simulink library "STMM"  (R2024a)
settings: Solver=VariableStepAuto  StartTime=0.0  StopTime=10.0  RelTol=1e-3
undefined symbols (not defined in the file or in its folder): raptor_xcp_function, StateCAN
libraries: Utilities x260, Raptor_lib x68, simulink x2
(part 3 of 3)

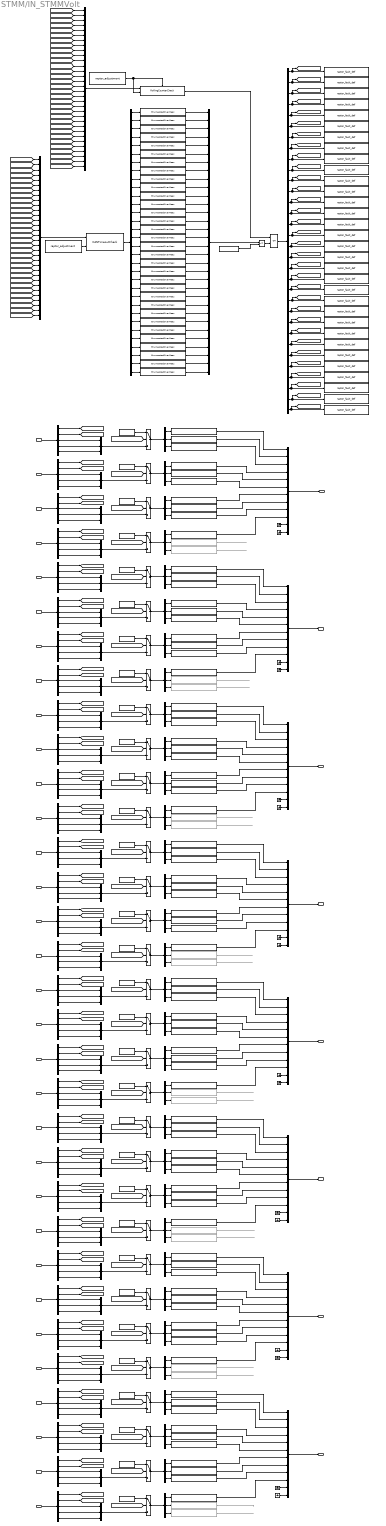
== system STMM/IN_STMMVolt ==
  IO_CAN2_332_Bus : Inport
  IO_CAN2_333_Bus : Inport  Port=2
  IO_CAN2_334_Bus : Inport  Port=3
  IO_CAN2_335_Bus : Inport  Port=4
  IO_CAN2_336_Bus : Inport  Port=5
  IO_CAN2_337_Bus : Inport  Port=6
  IO_CAN2_338_Bus : Inport  Port=7
  IO_CAN2_339_Bus : Inport  Port=8
  IO_CAN2_340_Bus : Inport  Port=9
  IO_CAN2_341_Bus : Inport  Port=10
  IO_CAN2_342_Bus : Inport  Port=11
  IO_CAN2_343_Bus : Inport  Port=12
  IO_CAN2_344_Bus : Inport  Port=13
  IO_CAN2_345_Bus : Inport  Port=14
  IO_CAN2_346_Bus : Inport  Port=15
  IO_CAN2_347_Bus : Inport  Port=16
  IO_CAN2_348_Bus : Inport  Port=17
  IO_CAN2_349_Bus : Inport  Port=18
  IO_CAN2_350_Bus : Inport  Port=19
  IO_CAN2_351_Bus : Inport  Port=20
  IO_CAN2_352_Bus : Inport  Port=21
  IO_CAN2_353_Bus : Inport  Port=22
  IO_CAN2_354_Bus : Inport  Port=23
  IO_CAN2_355_Bus : Inport  Port=24
  IO_CAN2_356_Bus : Inport  Port=25
  IO_CAN2_357_Bus : Inport  Port=26
  IO_CAN2_358_Bus : Inport  Port=27
  IO_CAN2_359_Bus : Inport  Port=28
  IO_CAN2_360_Bus : Inport  Port=29
  IO_CAN2_361_Bus : Inport  Port=30
  IO_CAN2_362_Bus : Inport  Port=31
  IO_CAN2_363_Bus : Inport  Port=32
  Bus Creator{,1..7} (8 alike) : BusCreator  Inputs=12
  Bus Selector : BusSelector  OutputSignals=Age,STMM_counterMsg332,STMM_segmentVolt100,STMM_segmentVolt101,STMM_segmentVolt102
  Bus Selector1 : BusSelector  OutputSignals=Age,STMM_counterMsg333,STMM_segmentVolt103,STMM_segmentVolt104,STMM_segmentVolt105
  Bus Selector10 : BusSelector  OutputSignals=Age,STMM_counterMsg342,STMM_segmentVolt306,STMM_segmentVolt307,STMM_segmentVolt308
  Bus Selector11 : BusSelector  OutputSignals=Age,STMM_counterMsg343,STMM_segmentVolt309,STMM_segmentVolt310,STMM_segmentVolt311
  Bus Selector12 : BusSelector  OutputSignals=Age,STMM_counterMsg344,STMM_segmentVolt400,STMM_segmentVolt401,STMM_segmentVolt402
  Bus Selector13 : BusSelector  OutputSignals=Age,STMM_counterMsg345,STMM_segmentVolt403,STMM_segmentVolt404,STMM_segmentVolt405
  Bus Selector14 : BusSelector  OutputSignals=Age,STMM_counterMsg346,STMM_segmentVolt406,STMM_segmentVolt407,STMM_segmentVolt408
  Bus Selector15 : BusSelector  OutputSignals=Age,STMM_counterMsg347,STMM_segmentVolt409,STMM_segmentVolt410,STMM_segmentVolt411
  Bus Selector16 : BusSelector  OutputSignals=Age,STMM_counterMsg348,STMM_segmentVolt500,STMM_segmentVolt501,STMM_segmentVolt502
  Bus Selector17 : BusSelector  OutputSignals=Age,STMM_counterMsg349,STMM_segmentVolt503,STMM_segmentVolt504,STMM_segmentVolt505
  Bus Selector18 : BusSelector  OutputSignals=Age,STMM_counterMsg350,STMM_segmentVolt506,STMM_segmentVolt507,STMM_segmentVolt508
  Bus Selector19 : BusSelector  OutputSignals=Age,STMM_counterMsg351,STMM_segmentVolt509,STMM_segmentVolt510,STMM_segmentVolt511
  Bus Selector2 : BusSelector  OutputSignals=Age,STMM_counterMsg334,STMM_segmentVolt106,STMM_segmentVolt107,STMM_segmentVolt108
  Bus Selector20 : BusSelector  OutputSignals=Age,STMM_counterMsg352,STMM_segmentVolt600,STMM_segmentVolt601,STMM_segmentVolt602
  Bus Selector21 : BusSelector  OutputSignals=Age,STMM_counterMsg353,STMM_segmentVolt603,STMM_segmentVolt604,STMM_segmentVolt605
  Bus Selector22 : BusSelector  OutputSignals=Age,STMM_counterMsg354,STMM_segmentVolt606,STMM_segmentVolt607,STMM_segmentVolt608
  Bus Selector23 : BusSelector  OutputSignals=Age,STMM_counterMsg355,STMM_segmentVolt609,STMM_segmentVolt610,STMM_segmentVolt611
  Bus Selector24 : BusSelector  OutputSignals=Age,STMM_counterMsg356,STMM_segmentVolt700,STMM_segmentVolt701,STMM_segmentVolt702
  Bus Selector25 : BusSelector  OutputSignals=Age,STMM_counterMsg357,STMM_segmentVolt703,STMM_segmentVolt704,STMM_segmentVolt705
  Bus Selector26 : BusSelector  OutputSignals=Age,STMM_counterMsg358,STMM_segmentVolt706,STMM_segmentVolt707,STMM_segmentVolt708
  Bus Selector27 : BusSelector  OutputSignals=Age,STMM_counterMsg359,STMM_segmentVolt709,STMM_segmentVolt710,STMM_segmentVolt711
  Bus Selector28 : BusSelector  OutputSignals=Age,STMM_counterMsg360,STMM_segmentVolt800,STMM_segmentVolt801,STMM_segmentVolt802
  Bus Selector29 : BusSelector  OutputSignals=Age,STMM_counterMsg361,STMM_segmentVolt803,STMM_segmentVolt804,STMM_segmentVolt805
  Bus Selector3 : BusSelector  OutputSignals=Age,STMM_counterMsg335,STMM_segmentVolt109,STMM_segmentVolt110,STMM_segmentVolt111
  Bus Selector30 : BusSelector  OutputSignals=Age,STMM_counterMsg362,STMM_segmentVolt806,STMM_segmentVolt807,STMM_segmentVolt808
  Bus Selector31 : BusSelector  OutputSignals=Age,STMM_counterMsg363,STMM_segmentVolt809,STMM_segmentVolt810,STMM_segmentVolt811
  Bus Selector4 : BusSelector  OutputSignals=Age,STMM_counterMsg336,STMM_segmentVolt200,STMM_segmentVolt201,STMM_segmentVolt202
  Bus Selector5 : BusSelector  OutputSignals=Age,STMM_counterMsg337,STMM_segmentVolt203,STMM_segmentVolt204,STMM_segmentVolt205
  Bus Selector6 : BusSelector  OutputSignals=Age,STMM_counterMsg338,STMM_segmentVolt206,STMM_segmentVolt207,STMM_segmentVolt208
  Bus Selector7 : BusSelector  OutputSignals=Age,STMM_counterMsg339,STMM_segmentVolt209,STMM_segmentVolt210,STMM_segmentVolt211
  Bus Selector8 : BusSelector  OutputSignals=Age,STMM_counterMsg340,STMM_segmentVolt300,STMM_segmentVolt301,STMM_segmentVolt302
  Bus Selector9 : BusSelector  OutputSignals=Age,STMM_counterMsg341,STMM_segmentVolt303,STMM_segmentVolt304,STMM_segmentVolt305
  CANTimeoutCheck : Utilities/CANTimeoutCheck
  Constant{1..32} (32 alike) : Constant  Value=int16(32767)
  Demux : Demux  Outputs=32
  Demux1 : Demux  Outputs=32
  Demux{2..33} (32 alike) : Demux  Outputs=3
  Enumerated Constant : simulink/Sources/Enumerated Constant  OutDataTypeStr=Enum: StateCAN  Value=StateCAN.Normal  SampleTime=inf
  EnumeratedOverMeas1 : Utilities/EnumeratedOverMeas  sigName='IN_CAN2_332_Status_en'  enumName='StateCAN'
  EnumeratedOverMeas10 : Utilities/EnumeratedOverMeas  sigName='IN_CAN2_341_Status_en'  enumName='StateCAN'
  EnumeratedOverMeas11 : Utilities/EnumeratedOverMeas  sigName='IN_CAN2_342_Status_en'  enumName='StateCAN'
  EnumeratedOverMeas12 : Utilities/EnumeratedOverMeas  sigName='IN_CAN2_343_Status_en'  enumName='StateCAN'
  EnumeratedOverMeas13 : Utilities/EnumeratedOverMeas  sigName='IN_CAN2_344_Status_en'  enumName='StateCAN'
  EnumeratedOverMeas14 : Utilities/EnumeratedOverMeas  sigName='IN_CAN2_345_Status_en'  enumName='StateCAN'
  EnumeratedOverMeas15 : Utilities/EnumeratedOverMeas  sigName='IN_CAN2_346_Status_en'  enumName='StateCAN'
  EnumeratedOverMeas16 : Utilities/EnumeratedOverMeas  sigName='IN_CAN2_347_Status_en'  enumName='StateCAN'
  EnumeratedOverMeas17 : Utilities/EnumeratedOverMeas  sigName='IN_CAN2_348_Status_en'  enumName='StateCAN'
  EnumeratedOverMeas18 : Utilities/EnumeratedOverMeas  sigName='IN_CAN2_349_Status_en'  enumName='StateCAN'
  EnumeratedOverMeas19 : Utilities/EnumeratedOverMeas  sigName='IN_CAN2_350_Status_en'  enumName='StateCAN'
  EnumeratedOverMeas2 : Utilities/EnumeratedOverMeas  sigName='IN_CAN2_333_Status_en'  enumName='StateCAN'
  EnumeratedOverMeas20 : Utilities/EnumeratedOverMeas  sigName='IN_CAN2_351_Status_en'  enumName='StateCAN'
  EnumeratedOverMeas21 : Utilities/EnumeratedOverMeas  sigName='IN_CAN2_352_Status_en'  enumName='StateCAN'
  EnumeratedOverMeas22 : Utilities/EnumeratedOverMeas  sigName='IN_CAN2_353_Status_en'  enumName='StateCAN'
  EnumeratedOverMeas23 : Utilities/EnumeratedOverMeas  sigName='IN_CAN2_354_Status_en'  enumName='StateCAN'
  EnumeratedOverMeas24 : Utilities/EnumeratedOverMeas  sigName='IN_CAN2_355_Status_en'  enumName='StateCAN'
  EnumeratedOverMeas25 : Utilities/EnumeratedOverMeas  sigName='IN_CAN2_356_Status_en'  enumName='StateCAN'
  EnumeratedOverMeas26 : Utilities/EnumeratedOverMeas  sigName='IN_CAN2_357_Status_en'  enumName='StateCAN'
  EnumeratedOverMeas27 : Utilities/EnumeratedOverMeas  sigName='IN_CAN2_358_Status_en'  enumName='StateCAN'
  EnumeratedOverMeas28 : Utilities/EnumeratedOverMeas  sigName='IN_CAN2_359_Status_en'  enumName='StateCAN'
  EnumeratedOverMeas29 : Utilities/EnumeratedOverMeas  sigName='IN_CAN2_360_Status_en'  enumName='StateCAN'
  EnumeratedOverMeas3 : Utilities/EnumeratedOverMeas  sigName='IN_CAN2_334_Status_en'  enumName='StateCAN'
  EnumeratedOverMeas30 : Utilities/EnumeratedOverMeas  sigName='IN_CAN2_361_Status_en'  enumName='StateCAN'
  EnumeratedOverMeas31 : Utilities/EnumeratedOverMeas  sigName='IN_CAN2_362_Status_en'  enumName='StateCAN'
  EnumeratedOverMeas32 : Utilities/EnumeratedOverMeas  sigName='IN_CAN2_363_Status_en'  enumName='StateCAN'
  EnumeratedOverMeas4 : Utilities/EnumeratedOverMeas  sigName='IN_CAN2_335_Status_en'  enumName='StateCAN'
  EnumeratedOverMeas5 : Utilities/EnumeratedOverMeas  sigName='IN_CAN2_336_Status_en'  enumName='StateCAN'
  EnumeratedOverMeas6 : Utilities/EnumeratedOverMeas  sigName='IN_CAN2_337_Status_en'  enumName='StateCAN'
  EnumeratedOverMeas7 : Utilities/EnumeratedOverMeas  sigName='IN_CAN2_338_Status_en'  enumName='StateCAN'
  EnumeratedOverMeas8 : Utilities/EnumeratedOverMeas  sigName='IN_CAN2_339_Status_en'  enumName='StateCAN'
  EnumeratedOverMeas9 : Utilities/EnumeratedOverMeas  sigName='IN_CAN2_340_Status_en'  enumName='StateCAN'
  Equal : RelationalOperator  Operator=~=  OutDataTypeStr=boolean  RndMeth=Simplest  InputSameDT=off
  Ground{,1..15} (16 alike) : Ground
  Mux{,1..31} (32 alike) : Mux  Inputs=3
  Mux32 : Mux  Inputs=32
  Mux33 : Mux  Inputs=32
  Mux34 : Mux  Inputs=32
  OR : Logic  Operator=OR  AllPortsSameDT=off  OutDataTypeStr=boolean
  OverMeas : Utilities/OverMeas  sigName='IN_SegmentVolt100_V'  minimum=-inf  maximum=inf
  OverMeas1 : Utilities/OverMeas  sigName='IN_SegmentVolt101_V'  minimum=-inf  maximum=inf
  OverMeas10 : Utilities/OverMeas  Commented=on  sigName='IN_SegmentTemp110_degC'  minimum=-inf  maximum=inf
  OverMeas11 : Utilities/OverMeas  Commented=on  sigName='IN_SegmentTemp111_degC'  minimum=-inf  maximum=inf
  OverMeas12 : Utilities/OverMeas  sigName='IN_SegmentVolt200_V'  minimum=-inf  maximum=inf
  OverMeas13 : Utilities/OverMeas  sigName='IN_SegmentVolt201_V'  minimum=-inf  maximum=inf
  OverMeas14 : Utilities/OverMeas  Commented=on  sigName='IN_SegmentTemp210_degC'  minimum=-inf  maximum=inf
  OverMeas15 : Utilities/OverMeas  Commented=on  sigName='IN_SegmentTemp211_degC'  minimum=-inf  maximum=inf
  OverMeas16 : Utilities/OverMeas  sigName='IN_SegmentVolt202_V'  minimum=-inf  maximum=inf
  OverMeas17 : Utilities/OverMeas  sigName='IN_SegmentVolt203_V'  minimum=-inf  maximum=inf
  OverMeas18 : Utilities/OverMeas  sigName='IN_SegmentVolt204_V'  minimum=-inf  maximum=inf
  OverMeas19 : Utilities/OverMeas  sigName='IN_SegmentVolt205_V'  minimum=-inf  maximum=inf
  OverMeas2 : Utilities/OverMeas  sigName='IN_SegmentVolt102_V'  minimum=-inf  maximum=inf
  OverMeas20 : Utilities/OverMeas  sigName='IN_SegmentVolt206_V'  minimum=-inf  maximum=inf
  OverMeas21 : Utilities/OverMeas  sigName='IN_SegmentVolt207_V'  minimum=-inf  maximum=inf
  OverMeas22 : Utilities/OverMeas  sigName='IN_SegmentVolt208_V'  minimum=-inf  maximum=inf
  OverMeas23 : Utilities/OverMeas  sigName='IN_SegmentVolt209_V'  minimum=-inf  maximum=inf
  OverMeas24 : Utilities/OverMeas  sigName='IN_SegmentVolt300_V'  minimum=-inf  maximum=inf
  OverMeas25 : Utilities/OverMeas  sigName='IN_SegmentVolt301_V'  minimum=-inf  maximum=inf
  OverMeas26 : Utilities/OverMeas  Commented=on  sigName='IN_SegmentTemp310_degC'  minimum=-inf  maximum=inf
  OverMeas27 : Utilities/OverMeas  Commented=on  sigName='IN_SegmentTemp311_degC'  minimum=-inf  maximum=inf
  OverMeas28 : Utilities/OverMeas  sigName='IN_SegmentVolt302_V'  minimum=-inf  maximum=inf
  OverMeas29 : Utilities/OverMeas  sigName='IN_SegmentVolt303_V'  minimum=-inf  maximum=inf
  OverMeas3 : Utilities/OverMeas  sigName='IN_SegmentVolt103_V'  minimum=-inf  maximum=inf
  OverMeas30 : Utilities/OverMeas  sigName='IN_SegmentVolt304_V'  minimum=-inf  maximum=inf
  OverMeas31 : Utilities/OverMeas  sigName='IN_SegmentVolt305_V'  minimum=-inf  maximum=inf
  OverMeas32 : Utilities/OverMeas  sigName='IN_SegmentVolt306_V'  minimum=-inf  maximum=inf
  OverMeas33 : Utilities/OverMeas  sigName='IN_SegmentVolt307_V'  minimum=-inf  maximum=inf
  OverMeas34 : Utilities/OverMeas  sigName='IN_SegmentVolt308_V'  minimum=-inf  maximum=inf
  OverMeas35 : Utilities/OverMeas  sigName='IN_SegmentVolt309_V'  minimum=-inf  maximum=inf
  OverMeas36 : Utilities/OverMeas  sigName='IN_SegmentVolt400_V'  minimum=-inf  maximum=inf
  OverMeas37 : Utilities/OverMeas  sigName='IN_SegmentVolt401_V'  minimum=-inf  maximum=inf
  OverMeas38 : Utilities/OverMeas  Commented=on  sigName='IN_SegmentTemp410_degC'  minimum=-inf  maximum=inf
  OverMeas39 : Utilities/OverMeas  Commented=on  sigName='IN_SegmentTemp411_degC'  minimum=-inf  maximum=inf
  OverMeas4 : Utilities/OverMeas  sigName='IN_SegmentVolt104_V'  minimum=-inf  maximum=inf
  OverMeas40 : Utilities/OverMeas  sigName='IN_SegmentVolt402_V'  minimum=-inf  maximum=inf
  OverMeas41 : Utilities/OverMeas  sigName='IN_SegmentVolt403_V'  minimum=-inf  maximum=inf
  OverMeas42 : Utilities/OverMeas  sigName='IN_SegmentVolt404_V'  minimum=-inf  maximum=inf
  OverMeas43 : Utilities/OverMeas  sigName='IN_SegmentVolt405_V'  minimum=-inf  maximum=inf
  OverMeas44 : Utilities/OverMeas  sigName='IN_SegmentVolt406_V'  minimum=-inf  maximum=inf
  OverMeas45 : Utilities/OverMeas  sigName='IN_SegmentVolt407_V'  minimum=-inf  maximum=inf
  OverMeas46 : Utilities/OverMeas  sigName='IN_SegmentVolt408_V'  minimum=-inf  maximum=inf
  OverMeas47 : Utilities/OverMeas  sigName='IN_SegmentVolt409_V'  minimum=-inf  maximum=inf
  OverMeas48 : Utilities/OverMeas  sigName='IN_SegmentVolt500_V'  minimum=-inf  maximum=inf
  OverMeas49 : Utilities/OverMeas  sigName='IN_SegmentVolt501_V'  minimum=-inf  maximum=inf
  OverMeas5 : Utilities/OverMeas  sigName='IN_SegmentVolt105_V'  minimum=-inf  maximum=inf
  OverMeas50 : Utilities/OverMeas  Commented=on  sigName='IN_SegmentTemp510_degC'  minimum=-inf  maximum=inf
  OverMeas51 : Utilities/OverMeas  Commented=on  sigName='IN_SegmentTemp511_degC'  minimum=-inf  maximum=inf
  OverMeas52 : Utilities/OverMeas  sigName='IN_SegmentVolt502_V'  minimum=-inf  maximum=inf
  OverMeas53 : Utilities/OverMeas  sigName='IN_SegmentVolt503_V'  minimum=-inf  maximum=inf
  OverMeas54 : Utilities/OverMeas  sigName='IN_SegmentVolt504_V'  minimum=-inf  maximum=inf
  OverMeas55 : Utilities/OverMeas  sigName='IN_SegmentVolt505_V'  minimum=-inf  maximum=inf
  OverMeas56 : Utilities/OverMeas  sigName='IN_SegmentVolt506_V'  minimum=-inf  maximum=inf
  OverMeas57 : Utilities/OverMeas  sigName='IN_SegmentVolt507_V'  minimum=-inf  maximum=inf
  OverMeas58 : Utilities/OverMeas  sigName='IN_SegmentVolt508_V'  minimum=-inf  maximum=inf
  OverMeas59 : Utilities/OverMeas  sigName='IN_SegmentVolt509_V'  minimum=-inf  maximum=inf
  OverMeas6 : Utilities/OverMeas  sigName='IN_SegmentVolt106_V'  minimum=-inf  maximum=inf
  OverMeas60 : Utilities/OverMeas  sigName='IN_SegmentVolt600_V'  minimum=-inf  maximum=inf
  OverMeas61 : Utilities/OverMeas  sigName='IN_SegmentVolt601_V'  minimum=-inf  maximum=inf
  OverMeas62 : Utilities/OverMeas  Commented=on  sigName='IN_SegmentTemp610_degC'  minimum=-inf  maximum=inf
  OverMeas63 : Utilities/OverMeas  Commented=on  sigName='IN_SegmentTemp611_degC'  minimum=-inf  maximum=inf
  OverMeas64 : Utilities/OverMeas  sigName='IN_SegmentVolt602_V'  minimum=-inf  maximum=inf
  OverMeas65 : Utilities/OverMeas  sigName='IN_SegmentVolt603_V'  minimum=-inf  maximum=inf
  OverMeas66 : Utilities/OverMeas  sigName='IN_SegmentVolt604_V'  minimum=-inf  maximum=inf
  OverMeas67 : Utilities/OverMeas  sigName='IN_SegmentVolt605_V'  minimum=-inf  maximum=inf
  OverMeas68 : Utilities/OverMeas  sigName='IN_SegmentVolt606_V'  minimum=-inf  maximum=inf
  OverMeas69 : Utilities/OverMeas  sigName='IN_SegmentVolt607_V'  minimum=-inf  maximum=inf
  OverMeas7 : Utilities/OverMeas  sigName='IN_SegmentVolt107_V'  minimum=-inf  maximum=inf
  OverMeas70 : Utilities/OverMeas  sigName='IN_SegmentVolt608_V'  minimum=-inf  maximum=inf
  OverMeas71 : Utilities/OverMeas  sigName='IN_SegmentVolt609_V'  minimum=-inf  maximum=inf
  OverMeas72 : Utilities/OverMeas  sigName='IN_SegmentVolt700_V'  minimum=-inf  maximum=inf
  OverMeas73 : Utilities/OverMeas  sigName='IN_SegmentVolt701_V'  minimum=-inf  maximum=inf
  OverMeas74 : Utilities/OverMeas  Commented=on  sigName='IN_SegmentTemp710_degC'  minimum=-inf  maximum=inf
  OverMeas75 : Utilities/OverMeas  Commented=on  sigName='IN_SegmentTemp711_degC'  minimum=-inf  maximum=inf
  OverMeas76 : Utilities/OverMeas  sigName='IN_SegmentVolt702_V'  minimum=-inf  maximum=inf
  OverMeas77 : Utilities/OverMeas  sigName='IN_SegmentVolt703_V'  minimum=-inf  maximum=inf
  OverMeas78 : Utilities/OverMeas  sigName='IN_SegmentVolt704_V'  minimum=-inf  maximum=inf
  OverMeas79 : Utilities/OverMeas  sigName='IN_SegmentVolt705_V'  minimum=-inf  maximum=inf
  OverMeas8 : Utilities/OverMeas  sigName='IN_SegmentVolt108_V'  minimum=-inf  maximum=inf
  OverMeas80 : Utilities/OverMeas  sigName='IN_SegmentVolt706_V'  minimum=-inf  maximum=inf
  OverMeas81 : Utilities/OverMeas  sigName='IN_SegmentVolt707_V'  minimum=-inf  maximum=inf
  OverMeas82 : Utilities/OverMeas  sigName='IN_SegmentVolt708_V'  minimum=-inf  maximum=inf
  OverMeas83 : Utilities/OverMeas  sigName='IN_SegmentVolt709_V'  minimum=-inf  maximum=inf
  OverMeas84 : Utilities/OverMeas  sigName='IN_SegmentVolt800_V'  minimum=-inf  maximum=inf
  OverMeas85 : Utilities/OverMeas  sigName='IN_SegmentVolt801_V'  minimum=-inf  maximum=inf
  OverMeas86 : Utilities/OverMeas  Commented=on  sigName='IN_SegmentTemp810_degC'  minimum=-inf  maximum=inf
  OverMeas87 : Utilities/OverMeas  Commented=on  sigName='IN_SegmentTemp811_degC'  minimum=-inf  maximum=inf
  OverMeas88 : Utilities/OverMeas  sigName='IN_SegmentVolt802_V'  minimum=-inf  maximum=inf
  OverMeas89 : Utilities/OverMeas  sigName='IN_SegmentVolt803_V'  minimum=-inf  maximum=inf
  OverMeas9 : Utilities/OverMeas  sigName='IN_SegmentVolt109_V'  minimum=-inf  maximum=inf
  OverMeas90 : Utilities/OverMeas  sigName='IN_SegmentVolt804_V'  minimum=-inf  maximum=inf
  OverMeas91 : Utilities/OverMeas  sigName='IN_SegmentVolt805_V'  minimum=-inf  maximum=inf
  OverMeas92 : Utilities/OverMeas  sigName='IN_SegmentVolt806_V'  minimum=-inf  maximum=inf
  OverMeas93 : Utilities/OverMeas  sigName='IN_SegmentVolt807_V'  minimum=-inf  maximum=inf
  OverMeas94 : Utilities/OverMeas  sigName='IN_SegmentVolt808_V'  minimum=-inf  maximum=inf
  OverMeas95 : Utilities/OverMeas  sigName='IN_SegmentVolt809_V'  minimum=-inf  maximum=inf
  RollingCounterCheck : Utilities/RollingCounterCheck
  Switch{1..32} (32 alike) : Switch  Criteria=u2 ~= 0  SaturateOnIntegerOverflow=off  InputSameDT=off
  raptor_adjustment : Raptor_lib/Data Storage/raptor_adjustment  paramName='IN_STMMVoltTOThresh_na'  nameSource=Parameter  initValue=200  dataType=uint32  storage=Calibration  calDispType=Number  calEnum={'False', 'True'}  calGain=1.0  calOffset=0.0  calMax=inf  calMin=-inf  calFormat='-1'  calUnit=''  calHelp=''  calAccess=1  calFunction=raptor_xcp_function(gcb)  calDispHeaders=off  calColHeaders={'Col1' 'Col2' 'Col3'}  calRowHeaders={'Row1' 'Row2' 'Row3'}
      settings: SourceProductName=Raptor
  raptor_adjustment1 : Raptor_lib/Data Storage/raptor_adjustment  paramName='IN_STMMVoltRollingCounterEnable_bool'  nameSource=Parameter  initValue=1  dataType=boolean  storage=Calibration  calDispType=Number  calEnum={'False', 'True'}  calGain=1.0  calOffset=0.0  calMax=inf  calMin=-inf  calFormat='-1'  calUnit=''  calHelp=''  calAccess=1  calFunction=raptor_xcp_function(gcb)  calDispHeaders=off  calColHeaders={'Col1' 'Col2' 'Col3'}  calRowHeaders={'Row1' 'Row2' 'Row3'}
      settings: SourceProductName=Raptor
  raptor_fault_def : Raptor_lib/Faults/raptor_fault_def  faultName='IN_CAN2_332_Fault'  persist=on  sticky=off  emisRelated=off  singleTrip=off  clearMethod=Standard  xLimit=25  yLimit=50  calEnable=on  addDisable=off  calAccess=1  calFunction='System | FaultManager'
      settings: SourceProductName=Raptor
  raptor_fault_def1 : Raptor_lib/Faults/raptor_fault_def  faultName='IN_CAN2_333_Fault'  persist=on  sticky=off  emisRelated=off  singleTrip=off  clearMethod=Standard  xLimit=25  yLimit=50  calEnable=on  addDisable=off  calAccess=1  calFunction='System | FaultManager'
      settings: SourceProductName=Raptor
  raptor_fault_def10 : Raptor_lib/Faults/raptor_fault_def  faultName='IN_CAN2_342_Fault'  persist=on  sticky=off  emisRelated=off  singleTrip=off  clearMethod=Standard  xLimit=25  yLimit=50  calEnable=on  addDisable=off  calAccess=1  calFunction='System | FaultManager'
      settings: SourceProductName=Raptor
  raptor_fault_def11 : Raptor_lib/Faults/raptor_fault_def  faultName='IN_CAN2_343_Fault'  persist=on  sticky=off  emisRelated=off  singleTrip=off  clearMethod=Standard  xLimit=25  yLimit=50  calEnable=on  addDisable=off  calAccess=1  calFunction='System | FaultManager'
      settings: SourceProductName=Raptor
  raptor_fault_def12 : Raptor_lib/Faults/raptor_fault_def  faultName='IN_CAN2_344_Fault'  persist=on  sticky=off  emisRelated=off  singleTrip=off  clearMethod=Standard  xLimit=25  yLimit=50  calEnable=on  addDisable=off  calAccess=1  calFunction='System | FaultManager'
      settings: SourceProductName=Raptor
  raptor_fault_def13 : Raptor_lib/Faults/raptor_fault_def  faultName='IN_CAN2_345_Fault'  persist=on  sticky=off  emisRelated=off  singleTrip=off  clearMethod=Standard  xLimit=25  yLimit=50  calEnable=on  addDisable=off  calAccess=1  calFunction='System | FaultManager'
      settings: SourceProductName=Raptor
  raptor_fault_def14 : Raptor_lib/Faults/raptor_fault_def  faultName='IN_CAN2_346_Fault'  persist=on  sticky=off  emisRelated=off  singleTrip=off  clearMethod=Standard  xLimit=25  yLimit=50  calEnable=on  addDisable=off  calAccess=1  calFunction='System | FaultManager'
      settings: SourceProductName=Raptor
  raptor_fault_def15 : Raptor_lib/Faults/raptor_fault_def  faultName='IN_CAN2_347_Fault'  persist=on  sticky=off  emisRelated=off  singleTrip=off  clearMethod=Standard  xLimit=25  yLimit=50  calEnable=on  addDisable=off  calAccess=1  calFunction='System | FaultManager'
      settings: SourceProductName=Raptor
  raptor_fault_def16 : Raptor_lib/Faults/raptor_fault_def  faultName='IN_CAN2_348_Fault'  persist=on  sticky=off  emisRelated=off  singleTrip=off  clearMethod=Standard  xLimit=25  yLimit=50  calEnable=on  addDisable=off  calAccess=1  calFunction='System | FaultManager'
      settings: SourceProductName=Raptor
  raptor_fault_def17 : Raptor_lib/Faults/raptor_fault_def  faultName='IN_CAN2_349_Fault'  persist=on  sticky=off  emisRelated=off  singleTrip=off  clearMethod=Standard  xLimit=25  yLimit=50  calEnable=on  addDisable=off  calAccess=1  calFunction='System | FaultManager'
      settings: SourceProductName=Raptor
  raptor_fault_def18 : Raptor_lib/Faults/raptor_fault_def  faultName='IN_CAN2_350_Fault'  persist=on  sticky=off  emisRelated=off  singleTrip=off  clearMethod=Standard  xLimit=25  yLimit=50  calEnable=on  addDisable=off  calAccess=1  calFunction='System | FaultManager'
      settings: SourceProductName=Raptor
  raptor_fault_def19 : Raptor_lib/Faults/raptor_fault_def  faultName='IN_CAN2_351_Fault'  persist=on  sticky=off  emisRelated=off  singleTrip=off  clearMethod=Standard  xLimit=25  yLimit=50  calEnable=on  addDisable=off  calAccess=1  calFunction='System | FaultManager'
      settings: SourceProductName=Raptor
  raptor_fault_def2 : Raptor_lib/Faults/raptor_fault_def  faultName='IN_CAN2_334_Fault'  persist=on  sticky=off  emisRelated=off  singleTrip=off  clearMethod=Standard  xLimit=25  yLimit=50  calEnable=on  addDisable=off  calAccess=1  calFunction='System | FaultManager'
      settings: SourceProductName=Raptor
  raptor_fault_def20 : Raptor_lib/Faults/raptor_fault_def  faultName='IN_CAN2_352_Fault'  persist=on  sticky=off  emisRelated=off  singleTrip=off  clearMethod=Standard  xLimit=25  yLimit=50  calEnable=on  addDisable=off  calAccess=1  calFunction='System | FaultManager'
      settings: SourceProductName=Raptor
  raptor_fault_def21 : Raptor_lib/Faults/raptor_fault_def  faultName='IN_CAN2_353_Fault'  persist=on  sticky=off  emisRelated=off  singleTrip=off  clearMethod=Standard  xLimit=25  yLimit=50  calEnable=on  addDisable=off  calAccess=1  calFunction='System | FaultManager'
      settings: SourceProductName=Raptor
  raptor_fault_def22 : Raptor_lib/Faults/raptor_fault_def  faultName='IN_CAN2_354_Fault'  persist=on  sticky=off  emisRelated=off  singleTrip=off  clearMethod=Standard  xLimit=25  yLimit=50  calEnable=on  addDisable=off  calAccess=1  calFunction='System | FaultManager'
      settings: SourceProductName=Raptor
  raptor_fault_def23 : Raptor_lib/Faults/raptor_fault_def  faultName='IN_CAN2_355_Fault'  persist=on  sticky=off  emisRelated=off  singleTrip=off  clearMethod=Standard  xLimit=25  yLimit=50  calEnable=on  addDisable=off  calAccess=1  calFunction='System | FaultManager'
      settings: SourceProductName=Raptor
  raptor_fault_def24 : Raptor_lib/Faults/raptor_fault_def  faultName='IN_CAN2_356_Fault'  persist=on  sticky=off  emisRelated=off  singleTrip=off  clearMethod=Standard  xLimit=25  yLimit=50  calEnable=on  addDisable=off  calAccess=1  calFunction='System | FaultManager'
      settings: SourceProductName=Raptor
  raptor_fault_def25 : Raptor_lib/Faults/raptor_fault_def  faultName='IN_CAN2_357_Fault'  persist=on  sticky=off  emisRelated=off  singleTrip=off  clearMethod=Standard  xLimit=25  yLimit=50  calEnable=on  addDisable=off  calAccess=1  calFunction='System | FaultManager'
      settings: SourceProductName=Raptor
  raptor_fault_def26 : Raptor_lib/Faults/raptor_fault_def  faultName='IN_CAN2_358_Fault'  persist=on  sticky=off  emisRelated=off  singleTrip=off  clearMethod=Standard  xLimit=25  yLimit=50  calEnable=on  addDisable=off  calAccess=1  calFunction='System | FaultManager'
      settings: SourceProductName=Raptor
  raptor_fault_def27 : Raptor_lib/Faults/raptor_fault_def  faultName='IN_CAN2_359_Fault'  persist=on  sticky=off  emisRelated=off  singleTrip=off  clearMethod=Standard  xLimit=25  yLimit=50  calEnable=on  addDisable=off  calAccess=1  calFunction='System | FaultManager'
      settings: SourceProductName=Raptor
  raptor_fault_def28 : Raptor_lib/Faults/raptor_fault_def  faultName='IN_CAN2_360_Fault'  persist=on  sticky=off  emisRelated=off  singleTrip=off  clearMethod=Standard  xLimit=25  yLimit=50  calEnable=on  addDisable=off  calAccess=1  calFunction='System | FaultManager'
      settings: SourceProductName=Raptor
  raptor_fault_def29 : Raptor_lib/Faults/raptor_fault_def  faultName='IN_CAN2_361_Fault'  persist=on  sticky=off  emisRelated=off  singleTrip=off  clearMethod=Standard  xLimit=25  yLimit=50  calEnable=on  addDisable=off  calAccess=1  calFunction='System | FaultManager'
      settings: SourceProductName=Raptor
  raptor_fault_def3 : Raptor_lib/Faults/raptor_fault_def  faultName='IN_CAN2_335_Fault'  persist=on  sticky=off  emisRelated=off  singleTrip=off  clearMethod=Standard  xLimit=25  yLimit=50  calEnable=on  addDisable=off  calAccess=1  calFunction='System | FaultManager'
      settings: SourceProductName=Raptor
  raptor_fault_def30 : Raptor_lib/Faults/raptor_fault_def  faultName='IN_CAN2_362_Fault'  persist=on  sticky=off  emisRelated=off  singleTrip=off  clearMethod=Standard  xLimit=25  yLimit=50  calEnable=on  addDisable=off  calAccess=1  calFunction='System | FaultManager'
      settings: SourceProductName=Raptor
  raptor_fault_def31 : Raptor_lib/Faults/raptor_fault_def  faultName='IN_CAN2_363_Fault'  persist=on  sticky=off  emisRelated=off  singleTrip=off  clearMethod=Standard  xLimit=25  yLimit=50  calEnable=on  addDisable=off  calAccess=1  calFunction='System | FaultManager'
      settings: SourceProductName=Raptor
  raptor_fault_def4 : Raptor_lib/Faults/raptor_fault_def  faultName='IN_CAN2_336_Fault'  persist=on  sticky=off  emisRelated=off  singleTrip=off  clearMethod=Standard  xLimit=25  yLimit=50  calEnable=on  addDisable=off  calAccess=1  calFunction='System | FaultManager'
      settings: SourceProductName=Raptor
  raptor_fault_def5 : Raptor_lib/Faults/raptor_fault_def  faultName='IN_CAN2_337_Fault'  persist=on  sticky=off  emisRelated=off  singleTrip=off  clearMethod=Standard  xLimit=25  yLimit=50  calEnable=on  addDisable=off  calAccess=1  calFunction='System | FaultManager'
      settings: SourceProductName=Raptor
  raptor_fault_def6 : Raptor_lib/Faults/raptor_fault_def  faultName='IN_CAN2_338_Fault'  persist=on  sticky=off  emisRelated=off  singleTrip=off  clearMethod=Standard  xLimit=25  yLimit=50  calEnable=on  addDisable=off  calAccess=1  calFunction='System | FaultManager'
      settings: SourceProductName=Raptor
  raptor_fault_def7 : Raptor_lib/Faults/raptor_fault_def  faultName='IN_CAN2_339_Fault'  persist=on  sticky=off  emisRelated=off  singleTrip=off  clearMethod=Standard  xLimit=25  yLimit=50  calEnable=on  addDisable=off  calAccess=1  calFunction='System | FaultManager'
      settings: SourceProductName=Raptor
  raptor_fault_def8 : Raptor_lib/Faults/raptor_fault_def  faultName='IN_CAN2_340_Fault'  persist=on  sticky=off  emisRelated=off  singleTrip=off  clearMethod=Standard  xLimit=25  yLimit=50  calEnable=on  addDisable=off  calAccess=1  calFunction='System | FaultManager'
      settings: SourceProductName=Raptor
  raptor_fault_def9 : Raptor_lib/Faults/raptor_fault_def  faultName='IN_CAN2_341_Fault'  persist=on  sticky=off  emisRelated=off  singleTrip=off  clearMethod=Standard  xLimit=25  yLimit=50  calEnable=on  addDisable=off  calAccess=1  calFunction='System | FaultManager'
      settings: SourceProductName=Raptor
  IN_Segment1Volt_Bus : Outport
  IN_Segment2Volt_Bus : Outport  Port=2
  IN_Segment3Volt_Bus : Outport  Port=3
  IN_Segment4Volt_Bus : Outport  Port=4
  IN_Segment5Volt_Bus : Outport  Port=5
  IN_Segment6Volt_Bus : Outport  Port=6
  IN_Segment7Volt_Bus : Outport  Port=7
  IN_Segment8Volt_Bus : Outport  Port=8
  wires:
  Ground15/1 -> Bus Creator7/12
  Ground14/1 -> Bus Creator7/11
  Ground13/1 -> Bus Creator6/12
  Ground12/1 -> Bus Creator6/11
  Ground11/1 -> Bus Creator5/12
  Ground10/1 -> Bus Creator5/11
  Ground9/1 -> Bus Creator4/12
  Ground8/1 -> Bus Creator4/11
  Ground7/1 -> Bus Creator3/12
  Ground6/1 -> Bus Creator3/11
  Ground5/1 -> Bus Creator2/12
  Ground4/1 -> Bus Creator2/11
  Ground3/1 -> Bus Creator1/12
  Ground2/1 -> Bus Creator1/11
  Ground1/1 -> Bus Creator/12
  Ground/1 -> Bus Creator/11
  OverMeas90/1 -> Bus Creator7/5  "IN_SegmentVolt804_V"
  Demux31/3 -> OverMeas91/1
  OverMeas92/1 -> Bus Creator7/7  "IN_SegmentVolt806_V"
  OverMeas91/1 -> Bus Creator7/6  "IN_SegmentVolt805_V"
  OverMeas87/1 -> ?  "IN_SegmentTemp811_degC"
  Demux33/3 -> OverMeas87/1
  Switch31/1 -> Demux32/1
  Switch29/1 -> Demux30/1
  Switch30/1 -> Demux31/1
  Switch32/1 -> Demux33/1
  OverMeas88/1 -> Bus Creator7/3  "IN_SegmentVolt802_V"
  Bus Creator7/1 -> IN_Segment8Volt_Bus/1  "IN_Segment8Volt_Bus"
  Demux32/3 -> OverMeas94/1
  OverMeas93/1 -> Bus Creator7/8  "IN_SegmentVolt807_V"
  Demux31/2 -> OverMeas90/1
  Demux33/2 -> OverMeas86/1
  OverMeas95/1 -> Bus Creator7/10  "IN_SegmentVolt809_V"
  Demux32/2 -> OverMeas93/1
  OverMeas85/1 -> Bus Creator7/2  "IN_SegmentVolt801_V"
  Demux32/1 -> OverMeas92/1
  OverMeas94/1 -> Bus Creator7/9  "IN_SegmentVolt808_V"
  OverMeas86/1 -> ?  "IN_SegmentTemp810_degC"
  Demux30/1 -> OverMeas84/1
  Demux33/1 -> OverMeas95/1
  Demux30/2 -> OverMeas85/1
  OverMeas84/1 -> Bus Creator7/1  "IN_SegmentVolt800_V"
  Demux30/3 -> OverMeas88/1
  Demux31/1 -> OverMeas89/1
  OverMeas89/1 -> Bus Creator7/4  "IN_SegmentVolt803_V"
  Demux29/2 -> OverMeas74/1
  Bus Creator6/1 -> IN_Segment7Volt_Bus/1  "IN_Segment7Volt_Bus"
  Demux27/2 -> OverMeas78/1
  OverMeas81/1 -> Bus Creator6/8  "IN_SegmentVolt707_V"
  Demux28/3 -> OverMeas82/1
  OverMeas76/1 -> Bus Creator6/3  "IN_SegmentVolt702_V"
  Demux28/1 -> OverMeas80/1
  OverMeas73/1 -> Bus Creator6/2  "IN_SegmentVolt701_V"
  OverMeas83/1 -> Bus Creator6/10  "IN_SegmentVolt709_V"
  Demux28/2 -> OverMeas81/1
  OverMeas82/1 -> Bus Creator6/9  "IN_SegmentVolt708_V"
  OverMeas77/1 -> Bus Creator6/4  "IN_SegmentVolt703_V"
  Demux27/1 -> OverMeas77/1
  Demux26/3 -> OverMeas76/1
  Demux26/2 -> OverMeas73/1
  OverMeas72/1 -> Bus Creator6/1  "IN_SegmentVolt700_V"
  Demux29/1 -> OverMeas83/1
  Demux26/1 -> OverMeas72/1
  OverMeas74/1 -> ?  "IN_SegmentTemp710_degC"
  Demux29/3 -> OverMeas75/1
  OverMeas79/1 -> Bus Creator6/6  "IN_SegmentVolt705_V"
  OverMeas80/1 -> Bus Creator6/7  "IN_SegmentVolt706_V"
  OverMeas78/1 -> Bus Creator6/5  "IN_SegmentVolt704_V"
  Demux27/3 -> OverMeas79/1
  OverMeas75/1 -> ?  "IN_SegmentTemp711_degC"
  Switch25/1 -> Demux26/1
  Switch27/1 -> Demux28/1
  Switch28/1 -> Demux29/1
  Switch26/1 -> Demux27/1
  Demux24/1 -> OverMeas68/1
  Demux25/2 -> OverMeas62/1
  Demux24/3 -> OverMeas70/1
  OverMeas65/1 -> Bus Creator5/4  "IN_SegmentVolt603_V"
  Demux24/2 -> OverMeas69/1
  OverMeas71/1 -> Bus Creator5/10  "IN_SegmentVolt609_V"
  OverMeas64/1 -> Bus Creator5/3  "IN_SegmentVolt602_V"
  Demux23/2 -> OverMeas66/1
  Bus Creator5/1 -> IN_Segment6Volt_Bus/1  "IN_Segment6Volt_Bus"
  OverMeas63/1 -> ?  "IN_SegmentTemp611_degC"
  OverMeas60/1 -> Bus Creator5/1  "IN_SegmentVolt600_V"
  Demux22/1 -> OverMeas60/1
  OverMeas62/1 -> ?  "IN_SegmentTemp610_degC"
  Demux23/1 -> OverMeas65/1
  Demux25/1 -> OverMeas71/1
  Demux22/2 -> OverMeas61/1
  Demux22/3 -> OverMeas64/1
  OverMeas69/1 -> Bus Creator5/8  "IN_SegmentVolt607_V"
  Switch23/1 -> Demux24/1
  Switch22/1 -> Demux23/1
  Switch21/1 -> Demux22/1
  Switch24/1 -> Demux25/1
  OverMeas67/1 -> Bus Creator5/6  "IN_SegmentVolt605_V"
  Demux25/3 -> OverMeas63/1
  Demux23/3 -> OverMeas67/1
  OverMeas70/1 -> Bus Creator5/9  "IN_SegmentVolt608_V"
  OverMeas61/1 -> Bus Creator5/2  "IN_SegmentVolt601_V"
  OverMeas66/1 -> Bus Creator5/5  "IN_SegmentVolt604_V"
  OverMeas68/1 -> Bus Creator5/7  "IN_SegmentVolt606_V"
  Demux19/1 -> OverMeas53/1
  Switch19/1 -> Demux20/1
  Switch17/1 -> Demux18/1
  OverMeas59/1 -> Bus Creator4/10  "IN_SegmentVolt509_V"
  Switch20/1 -> Demux21/1
  Switch18/1 -> Demux19/1
  OverMeas53/1 -> Bus Creator4/4  "IN_SegmentVolt503_V"
  Demux18/2 -> OverMeas49/1
  Bus Creator4/1 -> IN_Segment5Volt_Bus/1  "IN_Segment5Volt_Bus"
  Demux21/2 -> OverMeas50/1
  OverMeas51/1 -> ?  "IN_SegmentTemp511_degC"
  OverMeas57/1 -> Bus Creator4/8  "IN_SegmentVolt507_V"
  Demux18/3 -> OverMeas52/1
  OverMeas52/1 -> Bus Creator4/3  "IN_SegmentVolt502_V"
  OverMeas50/1 -> ?  "IN_SegmentTemp510_degC"
  OverMeas48/1 -> Bus Creator4/1  "IN_SegmentVolt500_V"
  Demux19/2 -> OverMeas54/1
  Demux20/2 -> OverMeas57/1
  Demux20/3 -> OverMeas58/1
  Demux21/1 -> OverMeas59/1
  OverMeas56/1 -> Bus Creator4/7  "IN_SegmentVolt506_V"
  Demux20/1 -> OverMeas56/1
  OverMeas55/1 -> Bus Creator4/6  "IN_SegmentVolt505_V"
  OverMeas49/1 -> Bus Creator4/2  "IN_SegmentVolt501_V"
  OverMeas54/1 -> Bus Creator4/5  "IN_SegmentVolt504_V"
  Demux19/3 -> OverMeas55/1
  OverMeas58/1 -> Bus Creator4/9  "IN_SegmentVolt508_V"
  Demux21/3 -> OverMeas51/1
  Demux18/1 -> OverMeas48/1
  Demux17/2 -> OverMeas38/1
  Bus Creator3/1 -> IN_Segment4Volt_Bus/1  "IN_Segment4Volt_Bus"
  OverMeas41/1 -> Bus Creator3/4  "IN_SegmentVolt403_V"
  Demux14/2 -> OverMeas37/1
  OverMeas47/1 -> Bus Creator3/10  "IN_SegmentVolt409_V"
  OverMeas39/1 -> ?  "IN_SegmentTemp411_degC"
  Demux14/1 -> OverMeas36/1
  Demux17/3 -> OverMeas39/1
  Demux15/3 -> OverMeas43/1
  OverMeas46/1 -> Bus Creator3/9  "IN_SegmentVolt408_V"
  OverMeas42/1 -> Bus Creator3/5  "IN_SegmentVolt404_V"
  OverMeas37/1 -> Bus Creator3/2  "IN_SegmentVolt401_V"
  OverMeas43/1 -> Bus Creator3/6  "IN_SegmentVolt405_V"
  Demux16/1 -> OverMeas44/1
  OverMeas44/1 -> Bus Creator3/7  "IN_SegmentVolt406_V"
  Demux17/1 -> OverMeas47/1
  OverMeas40/1 -> Bus Creator3/3  "IN_SegmentVolt402_V"
  Demux15/1 -> OverMeas41/1
  Switch16/1 -> Demux17/1
  Switch15/1 -> Demux16/1
  Demux16/3 -> OverMeas46/1
  Switch13/1 -> Demux14/1
  Switch14/1 -> Demux15/1
  OverMeas38/1 -> ?  "IN_SegmentTemp410_degC"
  OverMeas36/1 -> Bus Creator3/1  "IN_SegmentVolt400_V"
  Demux15/2 -> OverMeas42/1
  Demux16/2 -> OverMeas45/1
  Demux14/3 -> OverMeas40/1
  OverMeas45/1 -> Bus Creator3/8  "IN_SegmentVolt407_V"
  OverMeas29/1 -> Bus Creator2/4  "IN_SegmentVolt303_V"
  Demux13/2 -> OverMeas26/1
  Demux11/3 -> OverMeas31/1
  OverMeas30/1 -> Bus Creator2/5  "IN_SegmentVolt304_V"
  OverMeas35/1 -> Bus Creator2/10  "IN_SegmentVolt309_V"
  Demux10/1 -> OverMeas24/1
  Demux13/3 -> OverMeas27/1
  Switch9/1 -> Demux10/1
  OverMeas26/1 -> ?  "IN_SegmentTemp310_degC"
  Switch12/1 -> Demux13/1
  OverMeas24/1 -> Bus Creator2/1  "IN_SegmentVolt300_V"
  OverMeas32/1 -> Bus Creator2/7  "IN_SegmentVolt306_V"
  Demux13/1 -> OverMeas35/1
  Demux11/1 -> OverMeas29/1
  OverMeas28/1 -> Bus Creator2/3  "IN_SegmentVolt302_V"
  Switch11/1 -> Demux12/1
  Switch10/1 -> Demux11/1
  OverMeas31/1 -> Bus Creator2/6  "IN_SegmentVolt305_V"
  OverMeas33/1 -> Bus Creator2/8  "IN_SegmentVolt307_V"
  Demux12/3 -> OverMeas34/1
  Demux12/2 -> OverMeas33/1
  Demux11/2 -> OverMeas30/1
  OverMeas27/1 -> ?  "IN_SegmentTemp311_degC"
  Demux10/3 -> OverMeas28/1
  Demux10/2 -> OverMeas25/1
  Bus Creator2/1 -> IN_Segment3Volt_Bus/1  "IN_Segment3Volt_Bus"
  Demux12/1 -> OverMeas32/1
  OverMeas34/1 -> Bus Creator2/9  "IN_SegmentVolt308_V"
  OverMeas25/1 -> Bus Creator2/2  "IN_SegmentVolt301_V"
  Demux9/2 -> OverMeas14/1
  OverMeas16/1 -> Bus Creator1/3  "IN_SegmentVolt202_V"
  Demux7/3 -> OverMeas19/1
  OverMeas17/1 -> Bus Creator1/4  "IN_SegmentVolt203_V"
  Demux8/1 -> OverMeas20/1
  OverMeas20/1 -> Bus Creator1/7  "IN_SegmentVolt206_V"
  Demux9/3 -> OverMeas15/1
  Demux6/2 -> OverMeas13/1
  Demux7/1 -> OverMeas17/1
  Switch5/1 -> Demux7/1
  Demux6/3 -> OverMeas16/1
  OverMeas15/1 -> ?  "IN_SegmentTemp211_degC"
  OverMeas23/1 -> Bus Creator1/10  "IN_SegmentVolt209_V"
  Demux7/2 -> OverMeas18/1
  Switch7/1 -> Demux9/1
  Demux8/2 -> OverMeas21/1
  Demux8/3 -> OverMeas22/1
  OverMeas21/1 -> Bus Creator1/8  "IN_SegmentVolt207_V"
  OverMeas19/1 -> Bus Creator1/6  "IN_SegmentVolt205_V"
  OverMeas13/1 -> Bus Creator1/2  "IN_SegmentVolt201_V"
  OverMeas22/1 -> Bus Creator1/9  "IN_SegmentVolt208_V"
  OverMeas12/1 -> Bus Creator1/1  "IN_SegmentVolt200_V"
  OverMeas18/1 -> Bus Creator1/5  "IN_SegmentVolt204_V"
  Switch4/1 -> Demux6/1
  Demux6/1 -> OverMeas12/1
  Switch6/1 -> Demux8/1
  Bus Creator1/1 -> IN_Segment2Volt_Bus/1  "IN_Segment2Volt_Bus"
  OverMeas14/1 -> ?  "IN_SegmentTemp210_degC"
  Demux9/1 -> OverMeas23/1
  OverMeas11/1 -> ?  "IN_SegmentTemp111_degC"
  OverMeas10/1 -> ?  "IN_SegmentTemp110_degC"
  OverMeas9/1 -> Bus Creator/10  "IN_SegmentVolt109_V"
  OverMeas8/1 -> Bus Creator/9  "IN_SegmentVolt108_V"
  OverMeas7/1 -> Bus Creator/8  "IN_SegmentVolt107_V"
  OverMeas6/1 -> Bus Creator/7  "IN_SegmentVolt106_V"
  Demux5/3 -> OverMeas11/1
  Demux5/2 -> OverMeas10/1
  Demux5/1 -> OverMeas9/1
  Switch3/1 -> Demux5/1
  Demux4/3 -> OverMeas8/1
  Demux4/2 -> OverMeas7/1
  Demux4/1 -> OverMeas6/1
  Switch2/1 -> Demux4/1
  OverMeas5/1 -> Bus Creator/6  "IN_SegmentVolt105_V"
  OverMeas4/1 -> Bus Creator/5  "IN_SegmentVolt104_V"
  Demux3/3 -> OverMeas5/1
  Demux3/2 -> OverMeas4/1
  OverMeas3/1 -> Bus Creator/4  "IN_SegmentVolt103_V"
  Demux3/1 -> OverMeas3/1
  Switch1/1 -> Demux3/1
  Bus Creator/1 -> IN_Segment1Volt_Bus/1  "IN_Segment1Volt_Bus"
  OverMeas2/1 -> Bus Creator/3  "IN_SegmentVolt102_V"
  OverMeas1/1 -> Bus Creator/2  "IN_SegmentVolt101_V"
  OverMeas/1 -> Bus Creator/1  "IN_SegmentVolt100_V"
  Demux2/3 -> OverMeas2/1
  Demux2/2 -> OverMeas1/1
  Demux2/1 -> OverMeas/1
  Switch8/1 -> Demux2/1
  RollingCounterCheck/1 -> OR/1
  OR/1 -> Demux1/1
  raptor_adjustment1/1 -> RollingCounterCheck/Enable, RollingCounterCheck/2
  [IO_CAN2_363_cnt] -> Mux34/32
  [IO_CAN2_362_cnt] -> Mux34/31
  [IO_CAN2_361_cnt] -> Mux34/30
  [IO_CAN2_360_cnt] -> Mux34/29
  [IO_CAN2_359_cnt] -> Mux34/28
  [IO_CAN2_358_cnt] -> Mux34/27
  [IO_CAN2_357_cnt] -> Mux34/26
  [IO_CAN2_356_cnt] -> Mux34/25
  [IO_CAN2_355_cnt] -> Mux34/24
  [IO_CAN2_354_cnt] -> Mux34/23
  [IO_CAN2_353_cnt] -> Mux34/22
  [IO_CAN2_352_cnt] -> Mux34/21
  [IO_CAN2_351_cnt] -> Mux34/20
  [IO_CAN2_350_cnt] -> Mux34/19
  [IO_CAN2_349_cnt] -> Mux34/18
  [IO_CAN2_348_cnt] -> Mux34/17
  [IO_CAN2_347_cnt] -> Mux34/16
  [IO_CAN2_346_cnt] -> Mux34/15
  [IO_CAN2_345_cnt] -> Mux34/14
  [IO_CAN2_344_cnt] -> Mux34/13
  [IO_CAN2_343_cnt] -> Mux34/12
  [IO_CAN2_342_cnt] -> Mux34/11
  [IO_CAN2_341_cnt] -> Mux34/10
  [IO_CAN2_340_cnt] -> Mux34/9
  [IO_CAN2_339_cnt] -> Mux34/8
  [IO_CAN2_338_cnt] -> Mux34/7
  [IO_CAN2_337_cnt] -> Mux34/6
  [IO_CAN2_336_cnt] -> Mux34/5
  [IO_CAN2_335_cnt] -> Mux34/4
  [IO_CAN2_334_cnt] -> Mux34/3
  [IO_CAN2_333_cnt] -> Mux34/2
  [IO_CAN2_332_cnt] -> Mux34/1
  Mux34/1 -> RollingCounterCheck/1
  Mux31/1 -> Switch32/3
  Constant32/1 -> Switch32/1
  [IN_CAN2_363_Fault] -> Switch32/2
  Mux30/1 -> Switch31/3
  Constant31/1 -> Switch31/1
  [IN_CAN2_362_Fault] -> Switch31/2
  Mux29/1 -> Switch30/3
  Constant30/1 -> Switch30/1
  [IN_CAN2_361_Fault] -> Switch30/2
  Mux28/1 -> Switch29/3
  Constant29/1 -> Switch29/1
  [IN_CAN2_360_Fault] -> Switch29/2
  Constant28/1 -> Switch28/1
  [IN_CAN2_359_Fault] -> Switch28/2
  Mux27/1 -> Switch28/3
  Constant27/1 -> Switch27/1
  [IN_CAN2_358_Fault] -> Switch27/2
  Mux26/1 -> Switch27/3
  Constant26/1 -> Switch26/1
  [IN_CAN2_357_Fault] -> Switch26/2
  Mux25/1 -> Switch26/3
  Constant25/1 -> Switch25/1
  [IN_CAN2_356_Fault] -> Switch25/2
  Mux24/1 -> Switch25/3
  Constant24/1 -> Switch24/1
  [IN_CAN2_355_Fault] -> Switch24/2
  Mux23/1 -> Switch24/3
  Constant23/1 -> Switch23/1
  [IN_CAN2_354_Fault] -> Switch23/2
  Mux22/1 -> Switch23/3
  Constant22/1 -> Switch22/1
  [IN_CAN2_353_Fault] -> Switch22/2
  Mux21/1 -> Switch22/3
  Constant21/1 -> Switch21/1
  [IN_CAN2_352_Fault] -> Switch21/2
  Mux20/1 -> Switch21/3
  Constant20/1 -> Switch20/1
  [IN_CAN2_351_Fault] -> Switch20/2
  Mux19/1 -> Switch20/3
  Mux18/1 -> Switch19/3
  Constant19/1 -> Switch19/1
  [IN_CAN2_350_Fault] -> Switch19/2
  Mux17/1 -> Switch18/3
  Constant18/1 -> Switch18/1
  [IN_CAN2_349_Fault] -> Switch18/2
  Mux16/1 -> Switch17/3
  Constant17/1 -> Switch17/1
  [IN_CAN2_348_Fault] -> Switch17/2
  Mux15/1 -> Switch16/3
  Constant16/1 -> Switch16/1
  [IN_CAN2_347_Fault] -> Switch16/2
  Mux14/1 -> Switch15/3
  Constant15/1 -> Switch15/1
  [IN_CAN2_346_Fault] -> Switch15/2
  Mux13/1 -> Switch14/3
  Constant14/1 -> Switch14/1
  [IN_CAN2_345_Fault] -> Switch14/2
  Mux12/1 -> Switch13/3
  Constant13/1 -> Switch13/1
  [IN_CAN2_344_Fault] -> Switch13/2
  Mux11/1 -> Switch12/3
  Constant12/1 -> Switch12/1
  [IN_CAN2_343_Fault] -> Switch12/2
  Mux10/1 -> Switch11/3
  Constant11/1 -> Switch11/1
  [IN_CAN2_342_Fault] -> Switch11/2
  Mux9/1 -> Switch10/3
  Constant10/1 -> Switch10/1
  [IN_CAN2_341_Fault] -> Switch10/2
  Mux8/1 -> Switch9/3
  Constant9/1 -> Switch9/1
  [IN_CAN2_340_Fault] -> Switch9/2
  Mux7/1 -> Switch7/3
  Constant8/1 -> Switch7/1
  [IN_CAN2_339_Fault] -> Switch7/2
  Mux6/1 -> Switch6/3
  Constant7/1 -> Switch6/1
  [IN_CAN2_338_Fault] -> Switch6/2
  Mux5/1 -> Switch5/3
  Constant6/1 -> Switch5/1
  [IN_CAN2_337_Fault] -> Switch5/2
  Mux4/1 -> Switch4/3
  Constant5/1 -> Switch4/1
  [IN_CAN2_336_Fault] -> Switch4/2
  Mux3/1 -> Switch3/3
  Constant4/1 -> Switch3/1
  [IN_CAN2_335_Fault] -> Switch3/2
  Mux2/1 -> Switch2/3
  Constant3/1 -> Switch2/1
  [IN_CAN2_334_Fault] -> Switch2/2
  Mux1/1 -> Switch1/3
  Constant1/1 -> Switch1/1
  [IN_CAN2_333_Fault] -> Switch1/2
  Mux/1 -> Switch8/3
  [IN_CAN2_332_Fault] -> Switch8/2
  Constant2/1 -> Switch8/1
  Demux1/18 -> raptor_fault_def17/1, [IN_CAN2_349_Fault]
  Demux1/3 -> raptor_fault_def2/1, [IN_CAN2_334_Fault]
  Demux1/32 -> raptor_fault_def31/1, [IN_CAN2_363_Fault]
  Demux1/31 -> raptor_fault_def30/1, [IN_CAN2_362_Fault]
  Demux1/30 -> raptor_fault_def29/1, [IN_CAN2_361_Fault]
  Demux1/29 -> raptor_fault_def28/1, [IN_CAN2_360_Fault]
  Demux1/28 -> raptor_fault_def27/1, [IN_CAN2_359_Fault]
  Demux1/27 -> raptor_fault_def26/1, [IN_CAN2_358_Fault]
  Demux1/26 -> raptor_fault_def25/1, [IN_CAN2_357_Fault]
  Demux1/25 -> raptor_fault_def24/1, [IN_CAN2_356_Fault]
  Demux1/24 -> raptor_fault_def23/1, [IN_CAN2_355_Fault]
  Demux1/23 -> raptor_fault_def22/1, [IN_CAN2_354_Fault]
  Demux1/22 -> raptor_fault_def21/1, [IN_CAN2_353_Fault]
  Demux1/21 -> raptor_fault_def20/1, [IN_CAN2_352_Fault]
  Demux1/20 -> raptor_fault_def19/1, [IN_CAN2_351_Fault]
  Demux1/19 -> raptor_fault_def18/1, [IN_CAN2_350_Fault]
  Demux1/17 -> raptor_fault_def16/1, [IN_CAN2_348_Fault]
  Demux1/16 -> raptor_fault_def15/1, [IN_CAN2_347_Fault]
  Demux1/15 -> raptor_fault_def14/1, [IN_CAN2_346_Fault]
  Demux1/14 -> raptor_fault_def13/1, [IN_CAN2_345_Fault]
  Demux1/13 -> raptor_fault_def12/1, [IN_CAN2_344_Fault]
  Demux1/12 -> raptor_fault_def11/1, [IN_CAN2_343_Fault]
  Demux1/11 -> raptor_fault_def10/1, [IN_CAN2_342_Fault]
  Demux1/10 -> raptor_fault_def9/1, [IN_CAN2_341_Fault]
  Demux1/9 -> raptor_fault_def8/1, [IN_CAN2_340_Fault]
  Demux1/8 -> raptor_fault_def7/1, [IN_CAN2_339_Fault]
  Demux1/7 -> raptor_fault_def6/1, [IN_CAN2_338_Fault]
  Demux1/6 -> raptor_fault_def5/1, [IN_CAN2_337_Fault]
  Demux1/5 -> raptor_fault_def4/1, [IN_CAN2_336_Fault]
  Demux1/4 -> raptor_fault_def3/1, [IN_CAN2_335_Fault]
  Demux1/2 -> [IN_CAN2_333_Fault], raptor_fault_def1/1
  Demux1/1 -> [IN_CAN2_332_Fault], raptor_fault_def/1
  Equal/1 -> OR/2
  EnumeratedOverMeas32/1 -> Mux33/32  "IN_CAN2_363_Status_en"
  EnumeratedOverMeas31/1 -> Mux33/31  "IN_CAN2_362_Status_en"
  EnumeratedOverMeas30/1 -> Mux33/30  "IN_CAN2_361_Status_en"
  EnumeratedOverMeas29/1 -> Mux33/29  "IN_CAN2_360_Status_en"
  EnumeratedOverMeas28/1 -> Mux33/28  "IN_CAN2_359_Status_en"
  EnumeratedOverMeas27/1 -> Mux33/27  "IN_CAN2_358_Status_en"
  EnumeratedOverMeas26/1 -> Mux33/26  "IN_CAN2_357_Status_en"
  EnumeratedOverMeas25/1 -> Mux33/25  "IN_CAN2_356_Status_en"
  EnumeratedOverMeas24/1 -> Mux33/24  "IN_CAN2_355_Status_en"
  EnumeratedOverMeas23/1 -> Mux33/23  "IN_CAN2_354_Status_en"
  EnumeratedOverMeas22/1 -> Mux33/22  "IN_CAN2_353_Status_en"
  EnumeratedOverMeas21/1 -> Mux33/21  "IN_CAN2_352_Status_en"
  EnumeratedOverMeas20/1 -> Mux33/20  "IN_CAN2_351_Status_en"
  EnumeratedOverMeas19/1 -> Mux33/19  "IN_CAN2_350_Status_en"
  EnumeratedOverMeas18/1 -> Mux33/18  "IN_CAN2_349_Status_en"
  EnumeratedOverMeas17/1 -> Mux33/17  "IN_CAN2_348_Status_en"
  EnumeratedOverMeas16/1 -> Mux33/16  "IN_CAN2_347_Status_en"
  EnumeratedOverMeas15/1 -> Mux33/15  "IN_CAN2_346_Status_en"
  EnumeratedOverMeas14/1 -> Mux33/14  "IN_CAN2_345_Status_en"
  EnumeratedOverMeas13/1 -> Mux33/13  "IN_CAN2_344_Status_en"
  EnumeratedOverMeas12/1 -> Mux33/12  "IN_CAN2_343_Status_en"
  Demux/32 -> EnumeratedOverMeas32/1
  Demux/31 -> EnumeratedOverMeas31/1
  Demux/30 -> EnumeratedOverMeas30/1
  Demux/29 -> EnumeratedOverMeas29/1
  Demux/28 -> EnumeratedOverMeas28/1
  Demux/27 -> EnumeratedOverMeas27/1
  Demux/26 -> EnumeratedOverMeas26/1
  Demux/25 -> EnumeratedOverMeas25/1
  Demux/24 -> EnumeratedOverMeas24/1
  Demux/23 -> EnumeratedOverMeas23/1
  Demux/22 -> EnumeratedOverMeas22/1
  Demux/21 -> EnumeratedOverMeas21/1
  Demux/20 -> EnumeratedOverMeas20/1
  Demux/19 -> EnumeratedOverMeas19/1
  Demux/18 -> EnumeratedOverMeas18/1
  Demux/17 -> EnumeratedOverMeas17/1
  Demux/16 -> EnumeratedOverMeas16/1
  Demux/15 -> EnumeratedOverMeas15/1
  Demux/14 -> EnumeratedOverMeas14/1
  Demux/13 -> EnumeratedOverMeas13/1
  Demux/12 -> EnumeratedOverMeas12/1
  EnumeratedOverMeas11/1 -> Mux33/11  "IN_CAN2_342_Status_en"
  EnumeratedOverMeas10/1 -> Mux33/10  "IN_CAN2_341_Status_en"
  EnumeratedOverMeas9/1 -> Mux33/9  "IN_CAN2_340_Status_en"
  EnumeratedOverMeas8/1 -> Mux33/8  "IN_CAN2_339_Status_en"
  EnumeratedOverMeas7/1 -> Mux33/7  "IN_CAN2_338_Status_en"
  EnumeratedOverMeas6/1 -> Mux33/6  "IN_CAN2_337_Status_en"
  EnumeratedOverMeas5/1 -> Mux33/5  "IN_CAN2_336_Status_en"
  EnumeratedOverMeas4/1 -> Mux33/4  "IN_CAN2_335_Status_en"
  EnumeratedOverMeas3/1 -> Mux33/3  "IN_CAN2_334_Status_en"
  Demux/11 -> EnumeratedOverMeas11/1
  Demux/10 -> EnumeratedOverMeas10/1
  Demux/9 -> EnumeratedOverMeas9/1
  Demux/8 -> EnumeratedOverMeas8/1
  Demux/7 -> EnumeratedOverMeas7/1
  Demux/6 -> EnumeratedOverMeas6/1
  Demux/5 -> EnumeratedOverMeas5/1
  Demux/4 -> EnumeratedOverMeas4/1
  Demux/3 -> EnumeratedOverMeas3/1
  EnumeratedOverMeas2/1 -> Mux33/2  "IN_CAN2_333_Status_en"
  EnumeratedOverMeas1/1 -> Mux33/1  "IN_CAN2_332_Status_en"
  Demux/2 -> EnumeratedOverMeas2/1
  Demux/1 -> EnumeratedOverMeas1/1
  raptor_adjustment/1 -> CANTimeoutCheck/2
  Enumerated Constant/1 -> Equal/2
  Mux32/1 -> CANTimeoutCheck/1
  Mux33/1 -> Equal/1
  CANTimeoutCheck/1 -> Demux/1
  [IO_CAN2_363_Age] -> Mux32/32
  [IO_CAN2_362_Age] -> Mux32/31
  [IO_CAN2_361_Age] -> Mux32/30
  [IO_CAN2_360_Age] -> Mux32/29
  [IO_CAN2_359_Age] -> Mux32/28
  [IO_CAN2_358_Age] -> Mux32/27
  [IO_CAN2_357_Age] -> Mux32/26
  [IO_CAN2_356_Age] -> Mux32/25
  [IO_CAN2_355_Age] -> Mux32/24
  [IO_CAN2_354_Age] -> Mux32/23
  [IO_CAN2_353_Age] -> Mux32/22
  [IO_CAN2_352_Age] -> Mux32/21
  [IO_CAN2_351_Age] -> Mux32/20
  [IO_CAN2_350_Age] -> Mux32/19
  [IO_CAN2_349_Age] -> Mux32/18
  [IO_CAN2_348_Age] -> Mux32/17
  [IO_CAN2_347_Age] -> Mux32/16
  [IO_CAN2_346_Age] -> Mux32/15
  [IO_CAN2_345_Age] -> Mux32/14
  [IO_CAN2_344_Age] -> Mux32/13
  [IO_CAN2_343_Age] -> Mux32/12
  [IO_CAN2_342_Age] -> Mux32/11
  [IO_CAN2_341_Age] -> Mux32/10
  [IO_CAN2_340_Age] -> Mux32/9
  [IO_CAN2_339_Age] -> Mux32/8
  [IO_CAN2_338_Age] -> Mux32/7
  [IO_CAN2_337_Age] -> Mux32/6
  [IO_CAN2_336_Age] -> Mux32/5
  [IO_CAN2_335_Age] -> Mux32/4
  [IO_CAN2_334_Age] -> Mux32/3
  [IO_CAN2_333_Age] -> Mux32/2
  [IO_CAN2_332_Age] -> Mux32/1
  Bus Selector31/4 -> Mux31/2  "<STMM_segmentVolt810>"
  IO_CAN2_363_Bus/1 -> Bus Selector31/1
  Bus Selector31/5 -> Mux31/3  "<STMM_segmentVolt811>"
  Bus Selector31/3 -> Mux31/1  "<STMM_segmentVolt809>"
  Bus Selector31/2 -> [IO_CAN2_363_cnt]  "<STMM_counterMsg363>"
  Bus Selector31/1 -> [IO_CAN2_363_Age]  "<Age>"
  IO_CAN2_362_Bus/1 -> Bus Selector30/1
  Bus Selector30/3 -> Mux30/1  "<STMM_segmentVolt806>"
  Bus Selector30/4 -> Mux30/2  "<STMM_segmentVolt807>"
  Bus Selector30/2 -> [IO_CAN2_362_cnt]  "<STMM_counterMsg362>"
  Bus Selector30/5 -> Mux30/3  "<STMM_segmentVolt808>"
  Bus Selector30/1 -> [IO_CAN2_362_Age]  "<Age>"
  IO_CAN2_361_Bus/1 -> Bus Selector29/1
  Bus Selector29/1 -> [IO_CAN2_361_Age]  "<Age>"
  Bus Selector29/4 -> Mux29/2  "<STMM_segmentVolt804>"
  Bus Selector29/5 -> Mux29/3  "<STMM_segmentVolt805>"
  Bus Selector29/3 -> Mux29/1  "<STMM_segmentVolt803>"
  Bus Selector29/2 -> [IO_CAN2_361_cnt]  "<STMM_counterMsg361>"
  Bus Selector28/3 -> Mux28/1  "<STMM_segmentVolt800>"
  IO_CAN2_360_Bus/1 -> Bus Selector28/1
  Bus Selector28/2 -> [IO_CAN2_360_cnt]  "<STMM_counterMsg360>"
  Bus Selector28/4 -> Mux28/2  "<STMM_segmentVolt801>"
  Bus Selector28/1 -> [IO_CAN2_360_Age]  "<Age>"
  Bus Selector28/5 -> Mux28/3  "<STMM_segmentVolt802>"
  Bus Selector27/4 -> Mux27/2  "<STMM_segmentVolt710>"
  Bus Selector27/2 -> [IO_CAN2_359_cnt]  "<STMM_counterMsg359>"
  Bus Selector27/1 -> [IO_CAN2_359_Age]  "<Age>"
  IO_CAN2_359_Bus/1 -> Bus Selector27/1
  Bus Selector27/5 -> Mux27/3  "<STMM_segmentVolt711>"
  Bus Selector27/3 -> Mux27/1  "<STMM_segmentVolt709>"
  Bus Selector26/5 -> Mux26/3  "<STMM_segmentVolt708>"
  Bus Selector26/1 -> [IO_CAN2_358_Age]  "<Age>"
  IO_CAN2_358_Bus/1 -> Bus Selector26/1
  Bus Selector26/4 -> Mux26/2  "<STMM_segmentVolt707>"
  Bus Selector26/2 -> [IO_CAN2_358_cnt]  "<STMM_counterMsg358>"
  Bus Selector26/3 -> Mux26/1  "<STMM_segmentVolt706>"
  IO_CAN2_357_Bus/1 -> Bus Selector25/1
  Bus Selector25/5 -> Mux25/3  "<STMM_segmentVolt705>"
  Bus Selector25/3 -> Mux25/1  "<STMM_segmentVolt703>"
  Bus Selector25/1 -> [IO_CAN2_357_Age]  "<Age>"
  Bus Selector25/2 -> [IO_CAN2_357_cnt]  "<STMM_counterMsg357>"
  Bus Selector25/4 -> Mux25/2  "<STMM_segmentVolt704>"
  Bus Selector24/3 -> Mux24/1  "<STMM_segmentVolt700>"
  Bus Selector24/4 -> Mux24/2  "<STMM_segmentVolt701>"
  Bus Selector24/2 -> [IO_CAN2_356_cnt]  "<STMM_counterMsg356>"
  Bus Selector24/1 -> [IO_CAN2_356_Age]  "<Age>"
  IO_CAN2_356_Bus/1 -> Bus Selector24/1
  Bus Selector24/5 -> Mux24/3  "<STMM_segmentVolt702>"
  IO_CAN2_355_Bus/1 -> Bus Selector23/1
  Bus Selector23/2 -> [IO_CAN2_355_cnt]  "<STMM_counterMsg355>"
  Bus Selector23/4 -> Mux23/2  "<STMM_segmentVolt610>"
  Bus Selector23/3 -> Mux23/1  "<STMM_segmentVolt609>"
  Bus Selector23/5 -> Mux23/3  "<STMM_segmentVolt611>"
  Bus Selector23/1 -> [IO_CAN2_355_Age]  "<Age>"
  Bus Selector22/2 -> [IO_CAN2_354_cnt]  "<STMM_counterMsg354>"
  Bus Selector22/1 -> [IO_CAN2_354_Age]  "<Age>"
  Bus Selector22/5 -> Mux22/3  "<STMM_segmentVolt608>"
  Bus Selector22/4 -> Mux22/2  "<STMM_segmentVolt607>"
  Bus Selector22/3 -> Mux22/1  "<STMM_segmentVolt606>"
  IO_CAN2_354_Bus/1 -> Bus Selector22/1
  Bus Selector21/5 -> Mux21/3  "<STMM_segmentVolt605>"
  Bus Selector21/2 -> [IO_CAN2_353_cnt]  "<STMM_counterMsg353>"
  Bus Selector21/4 -> Mux21/2  "<STMM_segmentVolt604>"
  Bus Selector21/3 -> Mux21/1  "<STMM_segmentVolt603>"
  IO_CAN2_353_Bus/1 -> Bus Selector21/1
  Bus Selector21/1 -> [IO_CAN2_353_Age]  "<Age>"
  IO_CAN2_352_Bus/1 -> Bus Selector20/1
  Bus Selector20/2 -> [IO_CAN2_352_cnt]  "<STMM_counterMsg352>"
  Bus Selector20/4 -> Mux20/2  "<STMM_segmentVolt601>"
  Bus Selector20/5 -> Mux20/3  "<STMM_segmentVolt602>"
  Bus Selector20/3 -> Mux20/1  "<STMM_segmentVolt600>"
  Bus Selector20/1 -> [IO_CAN2_352_Age]  "<Age>"
  Bus Selector19/4 -> Mux19/2  "<STMM_segmentVolt510>"
  Bus Selector19/2 -> [IO_CAN2_351_cnt]  "<STMM_counterMsg351>"
  Bus Selector19/1 -> [IO_CAN2_351_Age]  "<Age>"
  Bus Selector19/5 -> Mux19/3  "<STMM_segmentVolt511>"
  Bus Selector19/3 -> Mux19/1  "<STMM_segmentVolt509>"
  IO_CAN2_351_Bus/1 -> Bus Selector19/1
  Bus Selector18/3 -> Mux18/1  "<STMM_segmentVolt506>"
  IO_CAN2_350_Bus/1 -> Bus Selector18/1
  Bus Selector18/1 -> [IO_CAN2_350_Age]  "<Age>"
  Bus Selector18/4 -> Mux18/2  "<STMM_segmentVolt507>"
  Bus Selector18/5 -> Mux18/3  "<STMM_segmentVolt508>"
  Bus Selector18/2 -> [IO_CAN2_350_cnt]  "<STMM_counterMsg350>"
  Bus Selector17/2 -> [IO_CAN2_349_cnt]  "<STMM_counterMsg349>"
  Bus Selector17/4 -> Mux17/2  "<STMM_segmentVolt504>"
  Bus Selector17/1 -> [IO_CAN2_349_Age]  "<Age>"
  Bus Selector17/5 -> Mux17/3  "<STMM_segmentVolt505>"
  IO_CAN2_349_Bus/1 -> Bus Selector17/1
  Bus Selector17/3 -> Mux17/1  "<STMM_segmentVolt503>"
  IO_CAN2_348_Bus/1 -> Bus Selector16/1
  Bus Selector16/3 -> Mux16/1  "<STMM_segmentVolt500>"
  Bus Selector16/5 -> Mux16/3  "<STMM_segmentVolt502>"
  Bus Selector16/2 -> [IO_CAN2_348_cnt]  "<STMM_counterMsg348>"
  Bus Selector16/1 -> [IO_CAN2_348_Age]  "<Age>"
  Bus Selector16/4 -> Mux16/2  "<STMM_segmentVolt501>"
  IO_CAN2_347_Bus/1 -> Bus Selector15/1
  Bus Selector15/2 -> [IO_CAN2_347_cnt]  "<STMM_counterMsg347>"
  Bus Selector15/3 -> Mux15/1  "<STMM_segmentVolt409>"
  Bus Selector15/1 -> [IO_CAN2_347_Age]  "<Age>"
  Bus Selector15/5 -> Mux15/3  "<STMM_segmentVolt411>"
  Bus Selector15/4 -> Mux15/2  "<STMM_segmentVolt410>"
  IO_CAN2_346_Bus/1 -> Bus Selector14/1
  Bus Selector14/4 -> Mux14/2  "<STMM_segmentVolt407>"
  Bus Selector14/3 -> Mux14/1  "<STMM_segmentVolt406>"
  Bus Selector14/5 -> Mux14/3  "<STMM_segmentVolt408>"
  Bus Selector14/1 -> [IO_CAN2_346_Age]  "<Age>"
  Bus Selector14/2 -> [IO_CAN2_346_cnt]  "<STMM_counterMsg346>"
  Bus Selector13/3 -> Mux13/1  "<STMM_segmentVolt403>"
  Bus Selector13/1 -> [IO_CAN2_345_Age]  "<Age>"
  Bus Selector13/2 -> [IO_CAN2_345_cnt]  "<STMM_counterMsg345>"
  Bus Selector13/5 -> Mux13/3  "<STMM_segmentVolt405>"
  Bus Selector13/4 -> Mux13/2  "<STMM_segmentVolt404>"
  IO_CAN2_345_Bus/1 -> Bus Selector13/1
  Bus Selector12/1 -> [IO_CAN2_344_Age]  "<Age>"
  Bus Selector12/2 -> [IO_CAN2_344_cnt]  "<STMM_counterMsg344>"
  Bus Selector12/4 -> Mux12/2  "<STMM_segmentVolt401>"
  IO_CAN2_344_Bus/1 -> Bus Selector12/1
  Bus Selector12/3 -> Mux12/1  "<STMM_segmentVolt400>"
  Bus Selector12/5 -> Mux12/3  "<STMM_segmentVolt402>"
  Bus Selector11/1 -> [IO_CAN2_343_Age]  "<Age>"
  Bus Selector11/2 -> [IO_CAN2_343_cnt]  "<STMM_counterMsg343>"
  Bus Selector11/4 -> Mux11/2  "<STMM_segmentVolt310>"
  Bus Selector11/5 -> Mux11/3  "<STMM_segmentVolt311>"
  Bus Selector11/3 -> Mux11/1  "<STMM_segmentVolt309>"
  IO_CAN2_343_Bus/1 -> Bus Selector11/1
  Bus Selector10/1 -> [IO_CAN2_342_Age]  "<Age>"
  IO_CAN2_342_Bus/1 -> Bus Selector10/1
  Bus Selector10/3 -> Mux10/1  "<STMM_segmentVolt306>"
  Bus Selector10/4 -> Mux10/2  "<STMM_segmentVolt307>"
  Bus Selector10/5 -> Mux10/3  "<STMM_segmentVolt308>"
  Bus Selector10/2 -> [IO_CAN2_342_cnt]  "<STMM_counterMsg342>"
  Bus Selector9/3 -> Mux9/1  "<STMM_segmentVolt303>"
  Bus Selector9/5 -> Mux9/3  "<STMM_segmentVolt305>"
  Bus Selector9/1 -> [IO_CAN2_341_Age]  "<Age>"
  Bus Selector9/4 -> Mux9/2  "<STMM_segmentVolt304>"
  IO_CAN2_341_Bus/1 -> Bus Selector9/1
  Bus Selector9/2 -> [IO_CAN2_341_cnt]  "<STMM_counterMsg341>"
  Bus Selector8/2 -> [IO_CAN2_340_cnt]  "<STMM_counterMsg340>"
  IO_CAN2_340_Bus/1 -> Bus Selector8/1
  Bus Selector8/3 -> Mux8/1  "<STMM_segmentVolt300>"
  Bus Selector8/5 -> Mux8/3  "<STMM_segmentVolt302>"
  Bus Selector8/1 -> [IO_CAN2_340_Age]  "<Age>"
  Bus Selector8/4 -> Mux8/2  "<STMM_segmentVolt301>"
  IO_CAN2_339_Bus/1 -> Bus Selector7/1
  Bus Selector7/5 -> Mux7/3  "<STMM_segmentVolt211>"
  Bus Selector7/4 -> Mux7/2  "<STMM_segmentVolt210>"
  Bus Selector7/1 -> [IO_CAN2_339_Age]  "<Age>"
  Bus Selector7/2 -> [IO_CAN2_339_cnt]  "<STMM_counterMsg339>"
  Bus Selector7/3 -> Mux7/1  "<STMM_segmentVolt209>"
  Bus Selector6/2 -> [IO_CAN2_338_cnt]  "<STMM_counterMsg338>"
  Bus Selector6/3 -> Mux6/1  "<STMM_segmentVolt206>"
  Bus Selector6/5 -> Mux6/3  "<STMM_segmentVolt208>"
  Bus Selector6/4 -> Mux6/2  "<STMM_segmentVolt207>"
  Bus Selector6/1 -> [IO_CAN2_338_Age]  "<Age>"
  IO_CAN2_338_Bus/1 -> Bus Selector6/1
  Bus Selector5/5 -> Mux5/3  "<STMM_segmentVolt205>"
  Bus Selector5/3 -> Mux5/1  "<STMM_segmentVolt203>"
  IO_CAN2_337_Bus/1 -> Bus Selector5/1
  Bus Selector5/1 -> [IO_CAN2_337_Age]  "<Age>"
  Bus Selector5/4 -> Mux5/2  "<STMM_segmentVolt204>"
  Bus Selector5/2 -> [IO_CAN2_337_cnt]  "<STMM_counterMsg337>"
  IO_CAN2_336_Bus/1 -> Bus Selector4/1
  Bus Selector4/4 -> Mux4/2  "<STMM_segmentVolt201>"
  Bus Selector4/3 -> Mux4/1  "<STMM_segmentVolt200>"
  Bus Selector4/5 -> Mux4/3  "<STMM_segmentVolt202>"
  Bus Selector4/2 -> [IO_CAN2_336_cnt]  "<STMM_counterMsg336>"
  Bus Selector4/1 -> [IO_CAN2_336_Age]  "<Age>"
  IO_CAN2_335_Bus/1 -> Bus Selector3/1
  Bus Selector3/4 -> Mux3/2  "<STMM_segmentVolt110>"
  Bus Selector3/3 -> Mux3/1  "<STMM_segmentVolt109>"
  Bus Selector3/1 -> [IO_CAN2_335_Age]  "<Age>"
  Bus Selector3/2 -> [IO_CAN2_335_cnt]  "<STMM_counterMsg335>"
  Bus Selector3/5 -> Mux3/3  "<STMM_segmentVolt111>"
  Bus Selector2/5 -> Mux2/3  "<STMM_segmentVolt108>"
  Bus Selector2/1 -> [IO_CAN2_334_Age]  "<Age>"
  Bus Selector2/2 -> [IO_CAN2_334_cnt]  "<STMM_counterMsg334>"
  Bus Selector2/4 -> Mux2/2  "<STMM_segmentVolt107>"
  Bus Selector2/3 -> Mux2/1  "<STMM_segmentVolt106>"
  IO_CAN2_334_Bus/1 -> Bus Selector2/1
  Bus Selector1/5 -> Mux1/3  "<STMM_segmentVolt105>"
  Bus Selector1/4 -> Mux1/2  "<STMM_segmentVolt104>"
  Bus Selector1/3 -> Mux1/1  "<STMM_segmentVolt103>"
  Bus Selector1/2 -> [IO_CAN2_333_cnt]  "<STMM_counterMsg333>"
  Bus Selector1/1 -> [IO_CAN2_333_Age]  "<Age>"
  IO_CAN2_333_Bus/1 -> Bus Selector1/1
  Bus Selector/5 -> Mux/3  "<STMM_segmentVolt102>"
  Bus Selector/4 -> Mux/2  "<STMM_segmentVolt101>"
  Bus Selector/3 -> Mux/1  "<STMM_segmentVolt100>"
  Bus Selector/2 -> [IO_CAN2_332_cnt]  "<STMM_counterMsg332>"
  Bus Selector/1 -> [IO_CAN2_332_Age]  "<Age>"
  IO_CAN2_332_Bus/1 -> Bus Selector/1
